simulink model "massSpringDamper"  (R2016a)
settings: Solver=VariableStepAuto  StartTime=0.0  StopTime=10.0  RelTol=1e-3
undefined symbols (not defined in the file or in its folder): const, ini
settings Model: Creator=s253428  LastModifiedBy=s253428

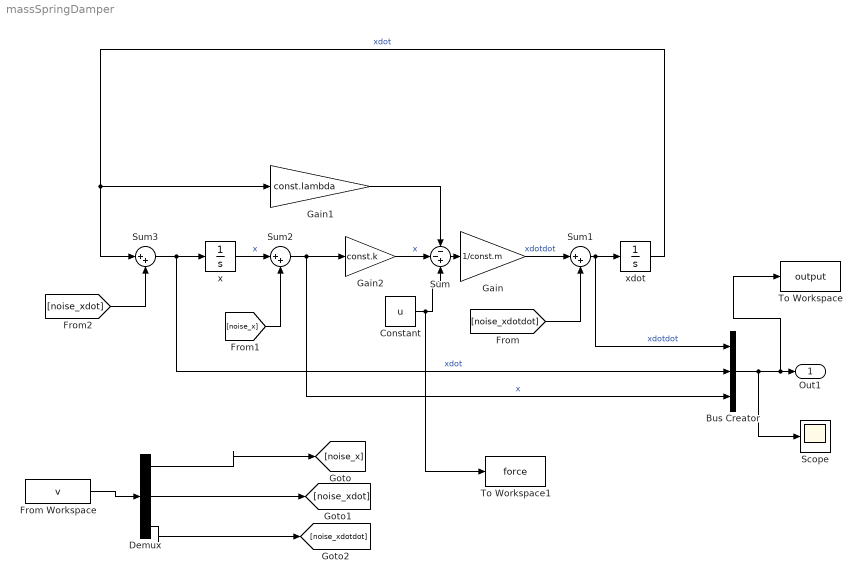
== system massSpringDamper ==
  Bus Creator : BusCreator  Inputs=3
  Constant : Constant  Value=u
  Demux : Demux  Outputs=3
  From Workspace : FromWorkspace  VariableName=v  SampleTime=0
  Gain : Gain  Gain=1/const.m
  Gain1 : Gain  Gain=const.lambda
  Gain2 : Gain  Gain=const.k
  Scope : Scope
  Sum : Sum  Inputs=--+
  Sum1 : Sum  Inputs=|++
  Sum2 : Sum  Inputs=|++
  Sum3 : Sum  Inputs=|++
  To Workspace : ToWorkspace  VariableName=output  SaveFormat=Timeseries  SampleTime=-1
  To Workspace1 : ToWorkspace  VariableName=force  SaveFormat=Timeseries  SampleTime=-1
  x : Integrator  InitialCondition=ini.x
  xdot : Integrator  InitialCondition=ini.xdot
  Out1 : Outport
  wires:
  Gain/1 -> Sum1/1  "xdotdot"
  Sum/1 -> Gain/1
  Constant/1 -> Sum/3, To Workspace1/1
  x/1 -> Sum2/1  "x"
  Gain1/1 -> Sum/1
  Bus Creator/1 -> Scope/1, To Workspace/1, Out1/1
  Sum1/1 -> Bus Creator/1, xdot/1  "xdotdot"
  Demux/3 -> [noise_xdotdot]
  [noise_xdotdot] -> Sum1/2
  Gain2/1 -> Sum/2  "x"
  Sum2/1 -> Gain2/1, Bus Creator/3  "x"
  [noise_x] -> Sum2/2
  xdot/1 -> Gain1/1, Sum3/1  "xdot"
  Sum3/1 -> Bus Creator/2, x/1  "xdot"
  [noise_xdot] -> Sum3/2
  Demux/2 -> [noise_xdot]
  Demux/1 -> [noise_x]
  From Workspace/1 -> Demux/1
